simulink model "Logistic"  (R2020b)
settings: Solver=ode45  StartTime=0.0  StopTime=30  RelTol=1e-6
settings Model: Creator=tian  LastModifiedBy=tian

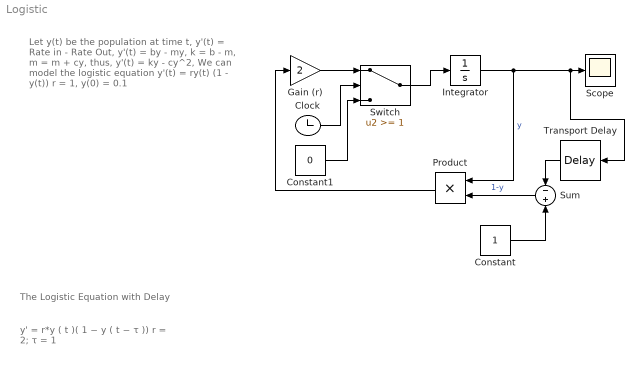
== system Logistic ==
  note: Let y(t) be the population at time t,
      |
      | y'(t) = Rate in - Rate Out,
      |
      | y'(t) = by - my,
      |
      | k = b - m,
      |
      | m = m + cy,
      |
      | thus,
      | y'(t) = ky - cy^2,
      |
      | We can model the logistic equation
      | y'(t) = ry(t) (1 - y(t))
      | r = 1, y(0) = 0.1
  note: The Logistic Equation with Delay
  note: y' = r*y ( t )( 1 − y ( t − τ ))
      | r = 2; τ = 1
  Clock : Clock
  Constant : Constant
  Constant1 : Constant  Value=0
  Gain (r) : Gain  Gain=2
  Integrator : Integrator  InitialCondition=2
  Product : Product
  Scope : Scope
  Sum : Sum  Inputs=-+
  Switch : Switch  Threshold=1
  Transport Delay : TransportDelay
  wires:
  Constant/1 -> Sum/2
  Sum/1 -> Product/2  "1-y"
  Integrator/1 -> Product/1, Transport Delay/1, Scope/1  "y"
  Product/1 -> Gain (r)/1
  Switch/1 -> Integrator/1
  Gain (r)/1 -> Switch/1
  Clock/1 -> Switch/2
  Constant1/1 -> Switch/3
  Transport Delay/1 -> Sum/1
